simulink model "Simulation_code"  (R2019b)
settings: Solver=ode4  StartTime=0.0  StopTime=10.0  FixedStep=ts  RelTol=1e-3
settings Model: Creator=auralius  LastModifiedBy=Anbazhagalan
settings DataIOCC: LimitDataPoints=on  SaveFormat=Array  ReturnWorkspaceOutputs=off
settings OptimizationCC: BlockReduction=off  BooleanDataType=off  LifeSpan=inf
settings DebuggingCC: SaveWithParameterizedLinksMsg=none  UnderspecifiedInitializationDetection=Classic  MergeDetectMultiDrivingBlocksExec=none  SignalResolutionControl=TryResolveAllWithWarning  SFUnexpectedBacktrackingDiag=warning  SFNoUnconditionalDefaultTransitionDiag=warning  SFExecutionAtInitializationDiag=none  ArithmeticOperatorsInVariantConditions=warning
settings HardwareCC: ProdBitPerPointer=32  ProdBitPerSizeT=32  ProdBitPerPtrDiffT=32  ProdLargestAtomicFloat=None  ProdIntDivRoundTo=Undefined  ProdEndianess=Unspecified  ProdWordSize=32  ProdHWDeviceType=32-bit Generic  TargetUnknown=on
settings ModelReferenceCC: PropagateSignalLabelsOutOfModel=off
settings SFSimCC: SimUseLocalCustomCode=off  CustomCodeUndefinedFunction=UseInterfaceOnly
settings RTWCC: RTWUseLocalCustomCode=off
settings CodeAppCC: StateflowObjectComments=on
settings GRTTargetCC: TargetLangStandard=C89/C90 (ANSI)  GeneratePreprocessorConditionals=Disable all
settings ConfigComp: CovMetricSettings=dw  CovHtmlReporting=on  CovSaveCumulativeToWorkspaceVar=on  CovSaveSingleToWorkspaceVar=on  CovExternalEMLEnable=off

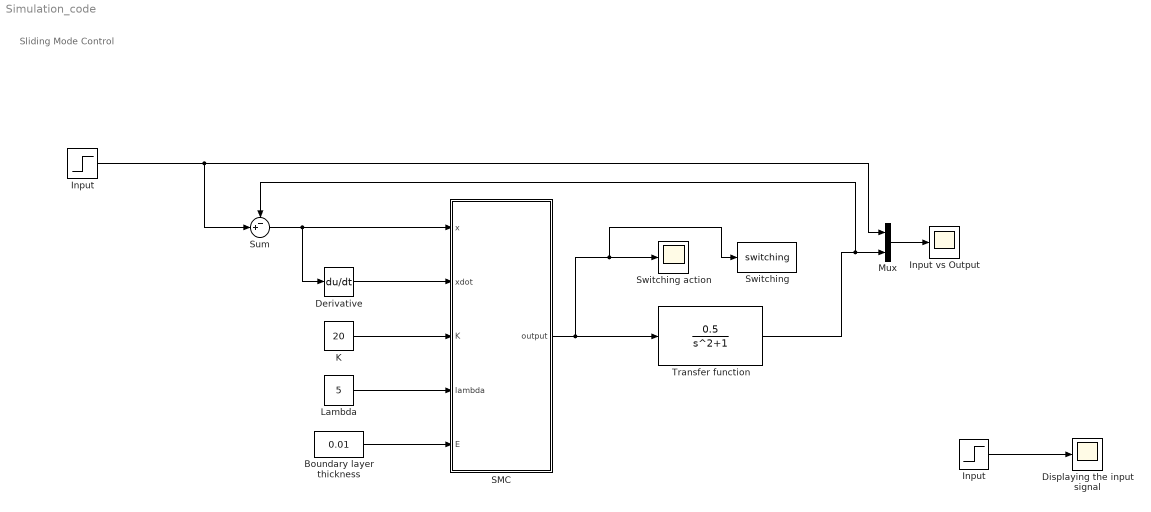
== system Simulation_code ==
  note: Sliding Mode Control
  Boundary layer thickness : Constant  Value=0.01
  Derivative : Derivative  CoefficientInTFapproximation=1
  Displaying the input signal : Scope
  Input : Step  SampleTime=0
  "Input " : Step  SampleTime=0
  Input vs Output : Scope
  K : Constant  Value=20
  Lambda : Constant  Value=5
  Mux : Mux  Inputs=2
  SMC : MATLAB Function  TreatAsAtomicUnit=on
  Sum : Sum  Inputs=-+|
  Switching : ToWorkspace  VariableName=switching  SampleTime=-1
  Switching action : Scope
  "Transfer function " : TransferFcn  Numerator=[0.5]  Denominator=[1 0 1]
  wires:
  Derivative/1 -> SMC/2(xdot)
  Sum/1 -> SMC/1(x), Derivative/1
  Lambda/1 -> SMC/4(lambda)
  K/1 -> SMC/3(K)
  Boundary layer thickness/1 -> SMC/5(E)
  Mux/1 -> Input vs Output/1
  SMC/1(output) -> "Transfer function "/1, Switching/1, Switching action/1
  "Input "/1 -> Mux/1, Sum/2
  "Transfer function "/1 -> Sum/1, Mux/2
  Input/1 -> Displaying the input signal/1

== matlab function Simulation_code/SMC ==
  data: x input; output output; xdot input; K input; lambda input; E input
function output = smc(x, xdot, K, lambda, E)
%#codegen

    s = lambda * x + xdot;
        
    if (abs(s) > E)    
        sat_s = sign(s);
    else
        sat_s = s/E;
    end
    
    output = -(xdot - K * sat_s);

end
